simulink model "autopilotcontrol"  (R2020a)
settings: Solver=VariableStepAuto  StartTime=0.0  StopTime=200  RelTol=1e-3
libraries: dspsrcs4 x4
settings Model: Creator=OZAN  LastModifiedBy=OZAN

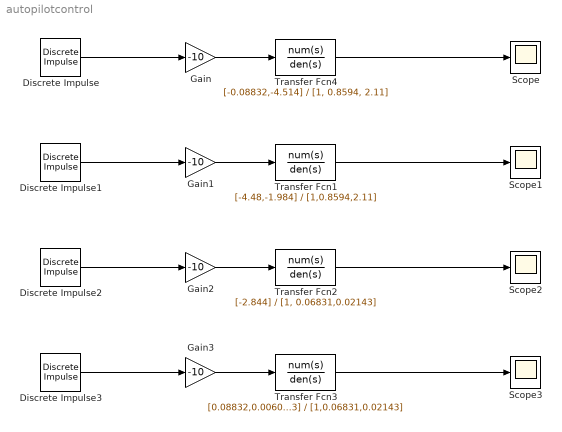
== system autopilotcontrol ==
  Discrete Impulse{,1..3} (4 alike) : dspsrcs4/Discrete  Impulse  Delay=0  SampleTime=1  FrameSample=1  OutputFrames=off  dataType=double  isSigned=on  wordLen=16  udDataType=sfix(16)  fracBitsMode=Best precision  numFracBits=15  OutDataTypeStr=double  LastOutDataTypeStr=double
  Gain{,1..3} (4 alike) : Gain  Gain=-10
  Scope{,1..3} (4 alike) : Scope
  Transfer Fcn1 : TransferFcn  Numerator=[-4.48,-1.984]  Denominator=[1,0.8594,2.11]
  Transfer Fcn2 : TransferFcn  Numerator=[-2.844]  Denominator=[1, 0.06831,0.02143]
  Transfer Fcn3 : TransferFcn  Numerator=[0.08832,0.006033]  Denominator=[1,0.06831,0.02143]
  Transfer Fcn4 : TransferFcn  Numerator=[-0.08832,-4.514]  Denominator=[1, 0.8594, 2.11]
  wires:
  Discrete Impulse/1 -> Gain/1
  Discrete Impulse1/1 -> Gain1/1
  Discrete Impulse2/1 -> Gain2/1
  Discrete Impulse3/1 -> Gain3/1
  Gain/1 -> Transfer Fcn4/1
  Gain1/1 -> Transfer Fcn1/1
  Gain2/1 -> Transfer Fcn2/1
  Gain3/1 -> Transfer Fcn3/1
  Transfer Fcn4/1 -> Scope/1
  Transfer Fcn1/1 -> Scope1/1
  Transfer Fcn2/1 -> Scope2/1
  Transfer Fcn3/1 -> Scope3/1
